simulink model "changeDetection"  (R2015a)
settings: configuration reference "AR_Drone_ConfigSet" (kept outside this file)
undefined symbols (not defined in the file or in its folder): Rec, SDTV, TotalBufferLength
libraries: visionconversions x2, ARdrone_video_lib x2, dspstat3 x1
settings Model: SimulationMode=external  CovSFcnEnable=off  ExtModeEnableFloating=off  ExtModeTrigDuration=120003  Creator=darenlee  LastModifiedBy=slovakad
settings ConfigSetRef: SourceLocation=Base Workspace

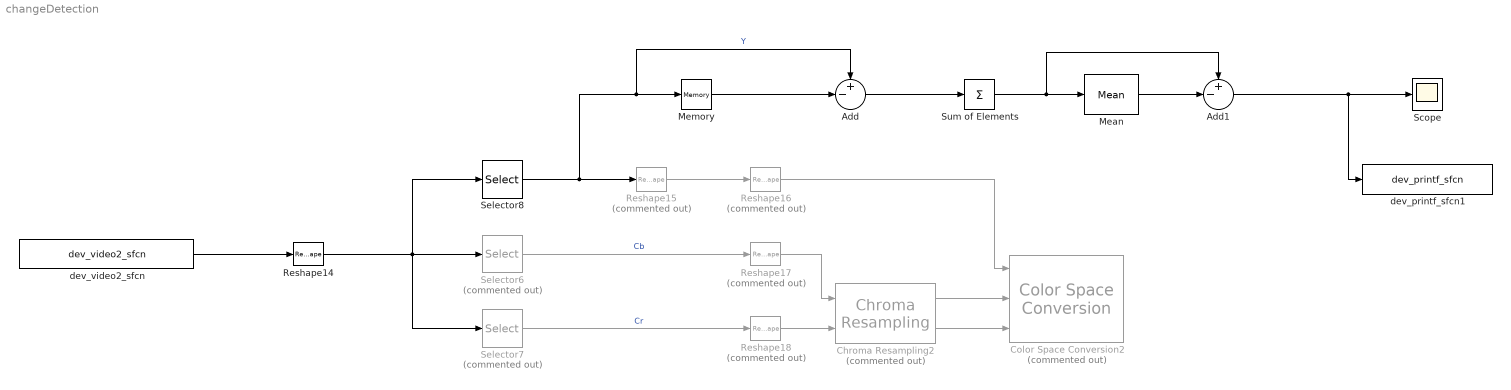
== system changeDetection ==
  Add : Sum  Inputs=+-|
  Add1 : Sum  Inputs=+-|
  Chroma Resampling2 : visionconversions/Chroma Resampling  Commented=on  resampling=4:2:2 to 4:4:4  interpolation=pixel replication  antialiasing=Default  hcoeff=[0.2 0.6 0.2]  vcoeff=[0.5 0.5]  isInputTransposed=on
  Color Space Conversion2 : visionconversions/Color Space  Conversion  Commented=on  conversion=Obsolete  conversionActive=Y'CbCr to R'G'B'  wp_str=D65  rec=Rec. 601 (SDTV)  sys=1125/60/2:1  imagePorts=Separate color signals
  Mean : dspstat3/Mean  run=on  reset_popup=None  directionMode=Each column  dimension=1  treatSBRowAsCol=off  roiEnable=off  roiType=Rectangles  roiPortion=Entire ROI  roiOutput=Individual statistics for each ROI  roiFlag=off  outputDataTypeStr=Inherit: Same as accumulator  outputLastDataTypeStr=Inherit: Same as accumulator  outputMin=[]  outputMax=[]  roundingMode=Floor  overflowMode=off
  Memory : Memory  X0=zeros(2,38400)  InheritSampleTime=on
  Reshape14 : Reshape  OutputDimensionality=Customize  OutputDimensions=[4 320*240*2/4]
  Reshape15 : Reshape  Commented=on  OutputDimensionality=Row vector (2-D)  OutputDimensions=[4 TotalBufferLength/4]
  Reshape16 : Reshape  Commented=on  OutputDimensionality=Customize  OutputDimensions=[320 240]
  Reshape17 : Reshape  Commented=on  OutputDimensionality=Customize  OutputDimensions=[320/2 240]
  Reshape18 : Reshape  Commented=on  OutputDimensionality=Customize  OutputDimensions=[320/2 240]
  Scope : Scope
      settings: YMin=-7e+06  YMax=8e+06
  Selector6 : Selector  Commented=on  NumberOfDimensions=2  InputPortWidth=3  IndexOptions=Index vector (dialog),Index vector (dialog)  Indices=1,[1:38400]  OutputSizes=1,1
  Selector7 : Selector  Commented=on  NumberOfDimensions=2  InputPortWidth=3  IndexOptions=Index vector (dialog),Index vector (dialog)  Indices=3,[1:38400]  OutputSizes=1,1
  Selector8 : Selector  NumberOfDimensions=2  InputPortWidth=3  IndexOptions=Index vector (dialog),Index vector (dialog)  Indices=[2 4],[1:38400]  OutputSizes=1,1
  Sum of Elements : Sum  Inputs=+  OutDataTypeStr=double
  dev_printf_sfcn1 : ARdrone_video_lib/dev_printf_sfcn  SFunctionSpec=ARpintf_Update(uint8 u1)  SampleTime=-1  ShowSpec=on
  dev_video2_sfcn : ARdrone_video_lib/dev_video2_sfcn  SFunctionSpec=videorabImage2(uint8 y1[153600])  SampleTime=1/25  ShowSpec=on
  wires:
  Sum of Elements/1 -> Mean/1, Add1/1
  Add/1 -> Sum of Elements/1
  Memory/1 -> Add/2
  Reshape17/1 -> Chroma Resampling2/1
  Reshape18/1 -> Chroma Resampling2/2
  Reshape16/1 -> Color Space Conversion2/1
  Reshape14/1 -> Selector8/1, Selector7/1, Selector6/1
  Selector6/1 -> Reshape17/1  "Cb"
  Chroma Resampling2/1 -> Color Space Conversion2/2
  Reshape15/1 -> Reshape16/1
  Chroma Resampling2/2 -> Color Space Conversion2/3
  dev_video2_sfcn/1 -> Reshape14/1
  Selector8/1 -> Reshape15/1, Memory/1, Add/1  "Y"
  Selector7/1 -> Reshape18/1  "Cr"
  Mean/1 -> Add1/2
  Add1/1 -> Scope/1, dev_printf_sfcn1/1
